simulink model "verify_lqr"  (R2018b)
settings: Solver=ode1  StartTime=0.0  StopTime=2  FixedStep=0.01  RelTol=1e-3
settings Model: Creator=Robert  LastModifiedBy=Robert

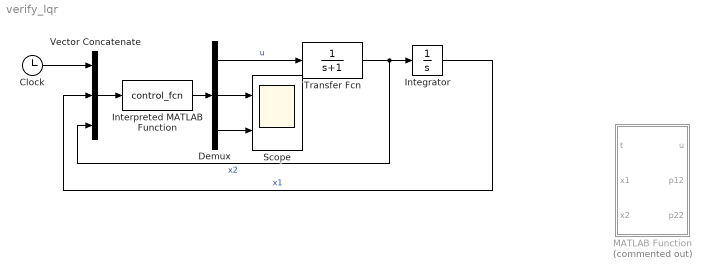
== system verify_lqr ==
  Clock : Clock
  Demux : Demux  Outputs=3
  Integrator : Integrator
  Interpreted MATLAB Function : MATLABFcn  MATLABFcn=control_fcn  OutputDimensions=3  Output1D=off
  MATLAB Function : MATLAB Function  Commented=on  TreatAsAtomicUnit=on
  Scope : Scope  NumInputPorts=2
  Transfer Fcn : TransferFcn  Denominator=[1 1]
  Vector Concatenate : Concatenate  NumInputs=3
  wires:
  Transfer Fcn/1 -> Vector Concatenate/3, Integrator/1  "x2"
  Demux/1 -> Transfer Fcn/1  "u"
  Integrator/1 -> Vector Concatenate/2  "x1"
  Demux/2 -> Scope/1
  Demux/3 -> Scope/2
  Clock/1 -> Vector Concatenate/1
  Vector Concatenate/1 -> Interpreted MATLAB Function/1
  Interpreted MATLAB Function/1 -> Demux/1

== matlab function verify_lqr/MATLAB Function ==
  data: t input; x1 input; u output; x2 input; p12 output; p22 output
function [u, p12, p22] = control(t, x1, x2)
coder.extrinsic('evalin')

controller = evalin('base', 'controller');

[u, p12, p22] = controller.control(t, [x1; x2]);
